simulink model "DAB_EPS_CL_model"  (R2024a)
settings: Solver=ode23t  StartTime=0.0  StopTime=0.07  RelTol=1e-3
undefined symbols (not defined in the file): ctrl, design, lut, N1, N2, spec
libraries: spsMosfetLib x8, spsVoltageMeasurementLib x5, spsCurrentMeasurementLib x4, spsSeriesRLCBranchLib x4, spsDCVoltageSourceLib x1, spsLinearTransformerLib x1, slpidlib x1, sps_lib x1
settings Model: Creator=abhik  LastModifiedBy=abhik

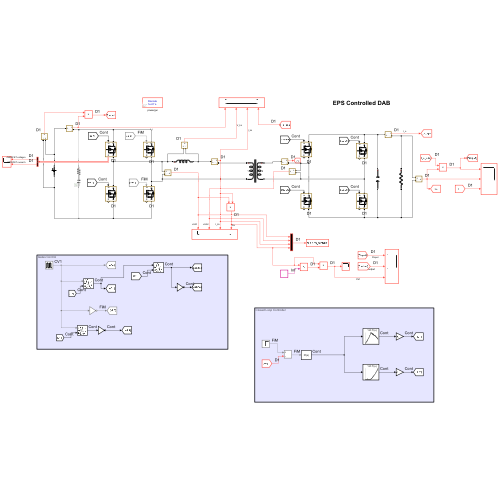
[thumbnail: Simulink's stored preview of the top-level diagram]
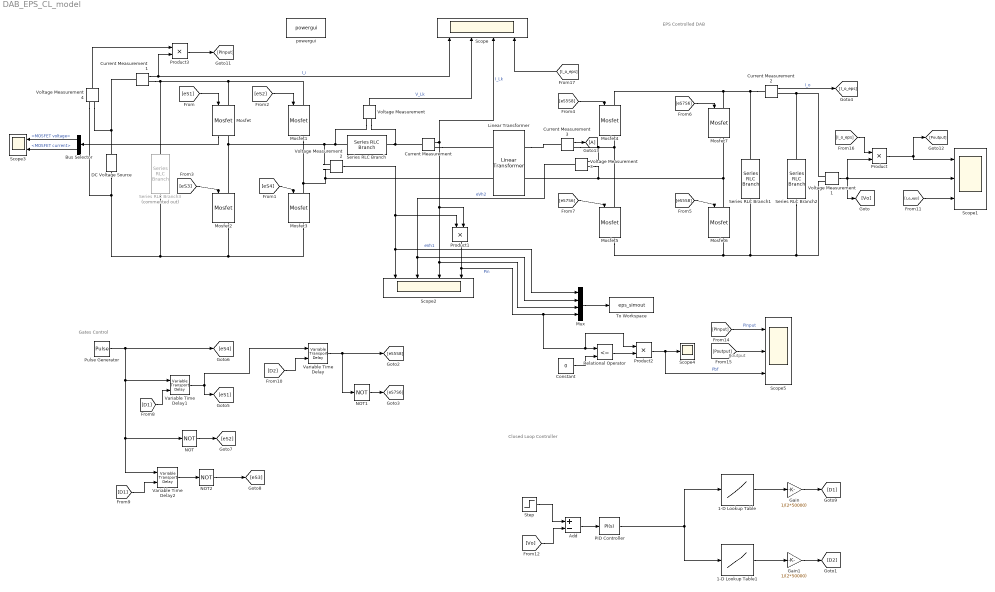
== system DAB_EPS_CL_model ==
  note: Poutput
  note: Closed Loop Controller
  note: Gates Control
  note: EPS Controlled DAB
  1-D Lookup Table : Lookup_n-D  NumberOfTableDimensions=1  BreakpointsForDimension1=lut.P_array  Table=lut.D1_table  ExtrapMethod=Clip  InternalRulePriority=Speed  RndMeth=Simplest
  1-D Lookup Table1 : Lookup_n-D  NumberOfTableDimensions=1  BreakpointsForDimension1=lut.P_array  Table=lut.D2_table  ExtrapMethod=Clip  InternalRulePriority=Speed  RndMeth=Simplest
  Add : Sum  Inputs=+-
  Bus Selector : BusSelector  OutputSignals=MOSFET voltage,MOSFET current
  Constant : Constant  Value=0
  Current Measurement{,1..3} (4 alike) : spsCurrentMeasurementLib/Current Measurement  PhasorSimulation=off  OutputType=Complex  PSBequivalent=0
  DC Voltage Source : spsDCVoltageSourceLib/DC Voltage Source  Amplitude=spec.V1  Measurements=None
  Gain : Gain  Gain=1/(2*50000)
  Gain1 : Gain  Gain=1/(2*50000)
  Goto13 : Goto
  Linear Transformer : spsLinearTransformerLib/Linear Transformer  UNITS=SI  NominalPower=[ 1.2*design.PN spec.fsw]  winding1=[N1 0 0]  winding2=[N2 0 0]  ThreeWindings=off  winding3=[3.15e+05 0.7938 0.084225]  RmLm=[1.0804e+06 2866]  Measurements=None  DataType=on
  Mosfet{,1..7} (8 alike) : spsMosfetLib/Mosfet  Ron=0.001  Lon=0  Rd=0.01  Vfd=0  IC=0  Rs=1e5  Cs=inf  Measurements=on
  Mux : Mux
  NOT : Logic  Operator=NOT  IconShape=distinctive  AllPortsSameDT=off  OutDataTypeStr=boolean
  NOT1 : Logic  Operator=NOT  IconShape=distinctive  AllPortsSameDT=off  OutDataTypeStr=boolean
  NOT2 : Logic  Operator=NOT  IconShape=distinctive  AllPortsSameDT=off  OutDataTypeStr=boolean
  PID Controller : slpidlib/PID Controller  Controller=PI  Form=Parallel  TimeDomain=Continuous-time  UseExternalTs=off  SampleTime=2e-5  IntegratorMethod=Forward Euler  FilterMethod=Forward Euler  ControllerParametersSource=internal  P=ctrl.Kp  I=ctrl.Ki  UseKiTs=off  D=0  UseExternalDerivativeSource=off  N=100  UseFilter=on  TunerSelectOption=Transfer Function Based (PID Tuner App)  InitialConditionSource=internal  InitialConditionForIntegrator=0  InitialConditionForFilter=0  DifferentiatorICPrevScaledInput=0  ExternalReset=none  TrackingMode=off  Kt=1  LimitOutput=off  SatLimitsSource=internal  UpperSaturationLimit=1000  LowerSaturationLimit=10  LinearizeAsGain=on  AntiWindupMode=clamping  Kb=1  LimitIntegrator=off  UpperIntegratorSaturationLimit=inf  LowerIntegratorSaturationLimit=-inf  POutMin=[]  POutMax=[]  IOutMin=[]  IOutMax=[]  DOutMin=[]  DOutMax=[]  NOutMin=[]  NOutMax=[]  SumOutMin=[]  SumOutMax=[]  SaturationOutMin=[]  SaturationOutMax=[]  PParamMin=[]  PParamMax=[]  IParamMin=[]  IParamMax=[]  DParamMin=[]  DParamMax=[]  NParamMin=[]  NParamMax=[]  KbParamMin=[]  KbParamMax=[]  KtParamMin=[]  KtParamMax=[]  KbOutMin=[]  KbOutMax=[]  KtOutMin=[]  KtOutMax=[]  IntegratorOutMin=[]  IntegratorOutMax=[]  FilterOutMin=[]  FilterOutMax=[]  SumI1OutMin=[]  SumI1OutMax=[]  SumI2OutMin=[]  SumI2OutMax=[]  SumI3OutMin=[]  SumI3OutMax=[]  SumI4OutMin=[]  SumI4OutMax=[]  SumDOutMin=[]  SumDOutMax=[]  DifferentiatorOutMin=[]  DifferentiatorOutMax=[]  FilterDiffOutCoefMin=[]  FilterDiffOutCoefMax=[]  ReciprocalOutMin=[]  ReciprocalOutMax=[]  SumDenOutMin=[]  SumDenOutMax=[]  SumNumOutMin=[]  SumNumOutMax=[]  DivideOutMin=[]  DivideOutMax=[]  UdiffTsProdOutMin=[]  UdiffTsProdOutMax=[]  NTsProdOutMin=[]  NTsProdOutMax=[]  UintegralTsProdOutMin=[]  UintegralTsProdOutMax=[]  UngainTsProdOutMin=[]  UngainTsProdOutMax=[]  ClampingZeroOutDataTypeStr=Inherit: Inherit via back propagation  ClampingZeroOutMin=[]  ClampingZeroOutMax=[]  FilterDenConstantOutDataTypeStr=Inherit: Inherit via back propagation  FilterDenConstantOutMin=[]  FilterDenConstantOutMax=[]  PCopyOutDataTypeStr=Inherit: Inherit via back propagation  PCopyOutMin=[]  PCopyOutMax=[]  NCopyOutDataTypeStr=Inherit: Inherit via back propagation  NCopyOutMin=[]  NCopyOutMax=[]  IntegratorContinuousStateAttributes=''  IntegratorStateMustResolveToSignalObject=off  IntegratorRTWStateStorageClass=Auto  FilterContinuousStateAttributes=''  FilterStateMustResolveToSignalObject=off  FilterRTWStateStorageClass=Auto  ParallelPVariant=InternalParameters  IdealPVariant=Disabled  IVariant=InternalParameters  DVariant=Disabled  IntegratorVariant=Continuous  SatVariant=Disabled  AWVariant=Passthrough  PCopyVariant=Disabled  TRVariant=Disabled  FdbkBlocksVariant=Forward  IdealPFdbkVariant=Disabled  SatFdbkVariant=Disabled  DerivativeFilterVariant=Disabled  NVariant=Disabled  NCopyVariant=Disabled_SignalSpec  FilterICVariant=Disabled  IntegratorICVariant=InternalICs  ExternalResetVariant=Disabled  TRSumVariant=Passthrough  SumFdbkVariant=Disabled  SumVariant=Sum_PI  TsampFilterVariant=InternalTs  TsampNgainVariant=Passthrough  TsampIntegralVariant=Disabled_SignalSpec  ExternalSaturationOutDataTypeStr=Inherit: Same as second input  DerivativeSourceVariant=Disabled
  Product{,1..3} (4 alike) : Product
  Pulse Generator : DiscretePulseGenerator  PulseType=Time based  Period=1/(spec.fsw)  PulseWidth=50
  Relational Operator : RelationalOperator  Operator=<=  OutDataTypeStr=boolean  RndMeth=Simplest  InputSameDT=off
  Scope : Scope  NumInputPorts=4
  Scope1 : Scope  NumInputPorts=3
  Scope2 : Scope  NumInputPorts=4
  Scope3 : Scope  NumInputPorts=2
  Scope4 : Scope
  Scope5 : Scope  NumInputPorts=3
  Series RLC Branch : spsSeriesRLCBranchLib/Series RLC Branch  LConnTagsString=__new0  RConnTagsString=__new0  BranchType=L  Resistance=1  Inductance=design.L  SetiL0=off  InitialCurrent=0  Capacitance=1e-6  Setx0=off  InitialVoltage=0  Measurements=None
  Series RLC Branch1 : spsSeriesRLCBranchLib/Series RLC Branch  LConnTagsString=__new0  RConnTagsString=__new0  BranchType=C  Resistance=1  Inductance=2.62e-6  SetiL0=off  InitialCurrent=0  Capacitance=spec.C  Setx0=off  InitialVoltage=0  Measurements=None
  Series RLC Branch2 : spsSeriesRLCBranchLib/Series RLC Branch  LConnTagsString=__new0  RConnTagsString=__new0  BranchType=R  Resistance=spec.R  Inductance=2.62e-6  SetiL0=off  InitialCurrent=0  Capacitance=3.13e-6  Setx0=off  InitialVoltage=0  Measurements=None
  Series RLC Branch3 : spsSeriesRLCBranchLib/Series RLC Branch  Commented=on  LConnTagsString=__new0  RConnTagsString=__new0  BranchType=RC  Resistance=0.66e-3  Inductance=1e-3  SetiL0=off  InitialCurrent=0  Capacitance=2.4e-4  Setx0=off  InitialVoltage=0  Measurements=None
  Step : Step  Time=0.03  Before=50  After=80  SampleTime=0
  To Workspace : ToWorkspace  VariableName=eps_simout  SaveFormat=Timeseries  SampleTime=-1
  Variable Time Delay : VariableTransportDelay  MaximumDelay=10
  Variable Time Delay1 : VariableTransportDelay  MaximumDelay=10
  Variable Time Delay2 : VariableTransportDelay  MaximumDelay=10
  Voltage Measurement{,1..4} (5 alike) : spsVoltageMeasurementLib/Voltage Measurement  PhasorSimulation=off  OutputType=Complex  PSBequivalent=0
  powergui : sps_lib/powergui  Priority=1  SimulationMode=Discrete  SampleTime=1e-7  frequency=60  Iterations=50  frequencyindice=0  Pbase=100e6  ErrMax=1e-4  UnitsV=kV  UnitsW=MW  buscounter=0  FunctionMessages=off  echomessages=off  EnableUseOfTLC=off  CurrentSourceSwitches=off  DisableSnubberDevices=off  DisableRonSwitches=off  DisableVfSwitches=off  DisplayEquations=off  AutomaticDiscreteSolvers=off  SolverType=Tustin/Backward Euler (TBE)  Interpol=off  ExternalGateDelay=off  methode=off  Ts=100  x0status=blocks  SPID=on  SwTol=0  HookPort=off  NonlinearTolerance=1e-4  nMaxIteration=100  ContinueOnMaxIteration=off  RestoreLinks=warning  ResistiveCurrentMeasurement=off  Frange=[0:2:500]  Ylog=off  Xlog=on  ShowGrid=off  save=off  variable=ZData  structure=0  ZoomFFT=off  StartTime=0.0  cycles=1  DisplayStyle=1  fundamental=60  FreqAxis=off  MaxFrequency=1000  frequencyindicesteady=1  RmsSteady=1  display=off
  wires:
  NOT/1 -> [eS2]
  Variable Time Delay2/1 -> NOT2/1
  Mux/1 -> To Workspace/1
  NOT1/1 -> [eS7S6]
  [eS7S6] -> Mosfet5/1
  Product1/1 -> Scope2/4, Mux/4, Relational Operator/1, Product2/1  "Pin"
  Voltage Measurement3/1 -> Scope2/2, Mux/2  "eVh2"
  Variable Time Delay1/1 -> [eS1], Variable Time Delay/1
  NOT2/1 -> [eS3]
  [eS4] -> Mosfet3/1
  Gain/1 -> [D1]
  Voltage Measurement1/1 -> [Vo], Scope1/2, Product/2
  [eS1] -> Mosfet/1
  [eS5S8] -> Mosfet4/1
  Gain1/1 -> [D2]
  [eS5S8] -> Mosfet6/1
  [D1] -> Variable Time Delay2/2
  [D1] -> Variable Time Delay1/2
  [eS2] -> Mosfet1/1
  Current Measurement/1 -> Product1/2, Scope2/3, Mux/3, Scope/3  "I_Lk"
  Voltage Measurement/1 -> Scope/2  "V_Lk"
  Voltage Measurement2/1 -> Scope2/1, Mux/1, Product1/1  "eVh1"
  Current Measurement1/1 -> Product3/2, Scope/1  "I_i"
  Current Measurement2/1 -> [I_o_eps]  "I_o"
  Pulse Generator/1 -> NOT/1, Variable Time Delay2/1, Variable Time Delay1/1, [eS4]
  [I_o_eps] -> Scope1/3
  [D2] -> Variable Time Delay/2
  [eS3] -> Mosfet2/1
  Variable Time Delay/1 -> [eS5S8], NOT1/1
  [eS7S6] -> Mosfet7/1
  Product/1 -> [Poutput], Scope1/1
  [Vo] -> Add/2
  Step/1 -> Add/1
  Add/1 -> PID Controller/1
  1-D Lookup Table/1 -> Gain/1
  1-D Lookup Table1/1 -> Gain1/1
  Mosfet/1 -> Bus Selector/1
  Bus Selector/1 -> Scope3/1  "<MOSFET voltage>"
  Bus Selector/2 -> Scope3/2  "<MOSFET current>"
  Constant/1 -> Relational Operator/2
  Relational Operator/1 -> Product2/2
  Product2/1 -> Scope4/1, Scope5/3  "Pbf"
  Voltage Measurement4/1 -> Product3/1
  Product3/1 -> [PInput]
  [PInput] -> Scope5/1  "Pinput"
  [Poutput] -> Scope5/2
  Current Measurement3/1 -> Goto13/1
  [I_o_eps] -> Product/1
  [I_o_eps] -> Scope/4
  PID Controller/1 -> 1-D Lookup Table1/1, 1-D Lookup Table/1
  connections:
  Voltage Measurement1/LConn2 -- Mosfet6/RConn1 -- Mosfet5/RConn1 -- Series RLC Branch1/RConn1 -- Series RLC Branch2/RConn1
  Voltage Measurement/LConn1 -- Voltage Measurement2/LConn1 -- Mosfet2/LConn1 -- Mosfet/RConn1 -- Series RLC Branch/LConn1
  Mosfet1/LConn1 -- Mosfet/LConn1 -- Series RLC Branch3/LConn1 -- Current Measurement1/RConn1
  DC Voltage Source/LConn1 -- Voltage Measurement4/LConn2 -- Mosfet2/RConn1 -- Mosfet3/RConn1 -- Series RLC Branch3/RConn1
  Linear Transformer/RConn2 -- Mosfet6/LConn1 -- Mosfet7/RConn1 -- Voltage Measurement3/LConn2
  Mosfet3/LConn1 -- Voltage Measurement2/LConn2 -- Linear Transformer/LConn2 -- Mosfet1/RConn1
  Voltage Measurement1/LConn1 -- Series RLC Branch2/LConn1 -- Current Measurement2/RConn1
  Mosfet4/RConn1 -- Mosfet5/LConn1 -- Voltage Measurement3/LConn1 -- Current Measurement3/RConn1
  Current Measurement2/LConn1 -- Mosfet4/LConn1 -- Mosfet7/LConn1 -- Series RLC Branch1/LConn1
  Series RLC Branch/RConn1 -- Current Measurement/LConn1 -- Voltage Measurement/LConn2
  Current Measurement/RConn1 -- Linear Transformer/LConn1
  DC Voltage Source/RConn1 -- Voltage Measurement4/LConn1 -- Current Measurement1/LConn1
  Linear Transformer/RConn1 -- Current Measurement3/LConn1
